simulink model "SEL_Model"  (R2022b)
settings: Solver=VariableStepAuto  StartTime=0.0  StopTime=10  RelTol=1e-3
model workspace (MAT data in the model file):
  QL = Simulink.Parameter
  QL.Value = 3000000
  QL.DataType = 'auto'
  QL.Complexity = 'real'
  QL.Dimensions = [1 1]
  RL = Simulink.Parameter
  RL.Value = 1560000000
  RL.DataType = 'auto'
  RL.Complexity = 'real'
  RL.Dimensions = [1 1]
  RQ = Simulink.Parameter
  RQ.Value = Simulink.data.Expression
  RQ.Value.ExpressionString = "RL/QL"
  RQ.DataType = 'auto'
  RQ.Complexity = 'real'
  RQ.Dimensions = -1
  Ts = Simulink.Parameter
  Ts.Value = 1e-07
  Ts.DataType = 'auto'
  Ts.Complexity = 'real'
  Ts.Dimensions = [1 1]
  a0 = Simulink.Parameter
  a0.Value = 1
  a0.DataType = 'auto'
  a0.Complexity = 'real'
  a0.Dimensions = [1 1]
  a1 = Simulink.Parameter
  a1.Value = -2
  a1.DataType = 'auto'
  a1.Complexity = 'real'
  a1.Dimensions = [1 1]
  a2 = Simulink.Parameter
  a2.Value = 1
  a2.DataType = 'auto'
  a2.Complexity = 'real'
  a2.Dimensions = [1 1]
  b0 = Simulink.Parameter
  b0.Value = -2.18e-09
  b0.DataType = 'auto'
  b0.Complexity = 'real'
  b0.Dimensions = [1 1]
  b1 = Simulink.Parameter
  b1.Value = -4.36e-09
  b1.DataType = 'auto'
  b1.Complexity = 'real'
  b1.Dimensions = [1 1]
  b2 = Simulink.Parameter
  b2.Value = -2.18e-09
  b2.DataType = 'auto'
  b2.Complexity = 'real'
  b2.Dimensions = [1 1]
  f0 = Simulink.Parameter
  f0.Value = 1300000000
  f0.DataType = 'auto'
  f0.Complexity = 'real'
  f0.Dimensions = [1 1]
  pi = Simulink.Parameter
  pi.Value = 3.1415926535
  pi.DataType = 'auto'
  pi.Complexity = 'real'
  pi.Dimensions = [1 1]
  w0 = Simulink.Parameter
  w0.Value = Simulink.data.Expression
  w0.Value.ExpressionString = "2*pi*390"
  w0.DataType = 'auto'
  w0.Complexity = 'real'
  w0.Dimensions = -1
  w_hbw = Simulink.Parameter
  w_hbw.Value = Simulink.data.Expression
  w_hbw.Value.ExpressionString = "2*pi*216"
  w_hbw.DataType = 'auto'
  w_hbw.Complexity = 'real'
  w_hbw.Dimensions = -1
settings Model: Creator=mliu  LastModifiedBy=mliu

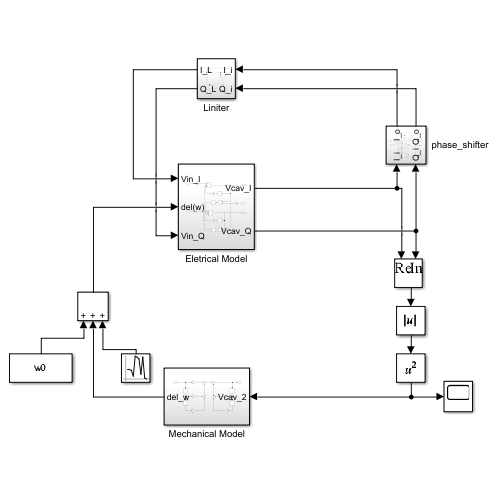
[thumbnail: Simulink's stored preview of the top-level diagram]
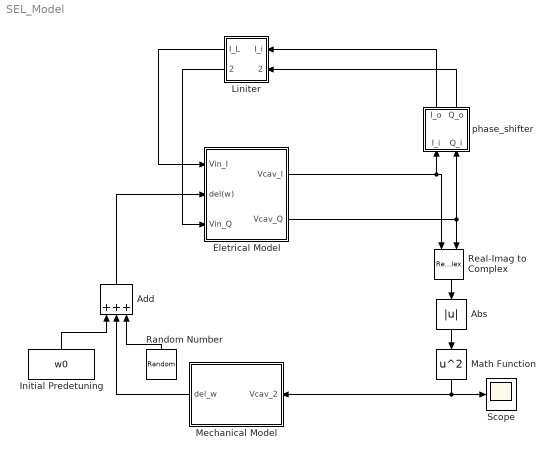
== system SEL_Model ==
  Abs : Abs  SaturateOnIntegerOverflow=off
  Add : Sum  Inputs=+++
  Eletrical Model : Subsystem
  Initial Predetuning : Constant  Value=w0
  Liniter : Subsystem
  Math Function : Math  Operator=square
  Mechanical Model : Subsystem
  Random Number : RandomNumber  SampleTime=0.1
  Real-Imag to Complex : RealImagToComplex
  Scope : Scope
  phase_shifter : Subsystem
  wires:
  Mechanical Model/1(del_w) -> Add/2
  Add/1 -> Eletrical Model/2(del(w))
  Initial Predetuning/1 -> Add/1
  Eletrical Model/1(Vcav_I) -> Real-Imag to Complex/1, phase_shifter/1(I_i)
  Eletrical Model/2(Vcav_Q) -> phase_shifter/2(Q_i), Real-Imag to Complex/2
  phase_shifter/1(I_o) -> Liniter/1(I_i)
  phase_shifter/2(Q_o) -> Liniter/2(Q_i)
  Liniter/2(Q_L) -> Eletrical Model/3(Vin_Q)
  Math Function/1 -> Scope/1, Mechanical Model/1(Vcav_2)
  Real-Imag to Complex/1 -> Abs/1
  Abs/1 -> Math Function/1
  Random Number/1 -> Add/3
  Liniter/1(I_L) -> Eletrical Model/1(Vin_I)

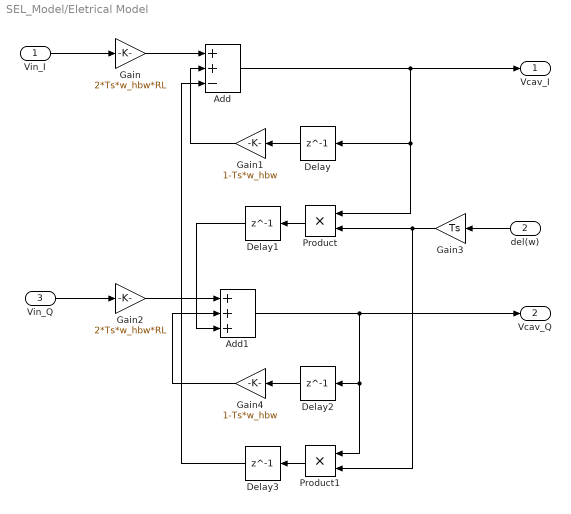
== system SEL_Model/Eletrical Model ==
  Vin_I : Inport
  del(w) : Inport  Port=2
  Vin_Q : Inport  Port=3
  Add : Sum  Inputs=++-
  Add1 : Sum  Inputs=+++
  Delay{,1..3} (4 alike) : Delay  DelayLength=1  InitialCondition=0
  Gain : Gain  Gain=2*Ts*w_hbw*RL
  Gain1 : Gain  Gain=1-Ts*w_hbw
  Gain2 : Gain  Gain=2*Ts*w_hbw*RL
  Gain3 : Gain  Gain=Ts
  Gain4 : Gain  Gain=1-Ts*w_hbw
  Product : Product
  Product1 : Product
  Vcav_I : Outport
  Vcav_Q : Outport  Port=2
  wires:
  Delay/1 -> Gain1/1
  Gain/1 -> Add/1
  Gain3/1 -> Product1/2, Product/2
  Add1/1 -> Vcav_Q/1, Product1/1, Delay2/1
  Add/1 -> Vcav_I/1, Product/1, Delay/1
  Delay1/1 -> Add1/3
  Product/1 -> Delay1/1
  Vin_Q/1 -> Gain2/1
  Vin_I/1 -> Gain/1
  Gain2/1 -> Add1/1
  Product1/1 -> Delay3/1
  Gain1/1 -> Add/2
  Delay2/1 -> Gain4/1
  Delay3/1 -> Add/3
  del(w)/1 -> Gain3/1
  Gain4/1 -> Add1/2

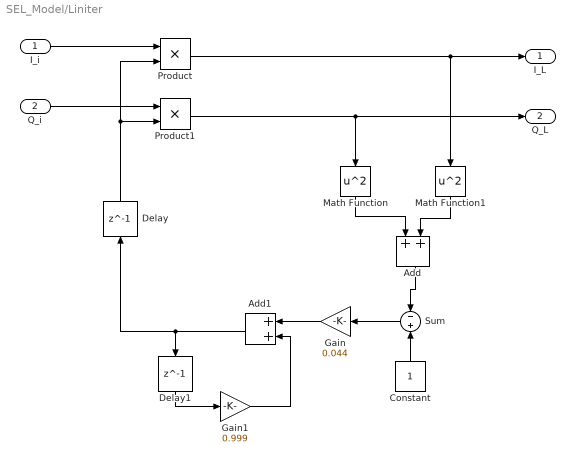
== system SEL_Model/Liniter ==
  I_i : Inport
  Q_i : Inport  Port=2
  Add : Sum
  Add1 : Sum
  Constant : Constant
  Delay : Delay  DelayLength=1  InitialCondition=0
  Delay1 : Delay  DelayLength=1  InitialCondition=0
  Gain : Gain  Gain=0.044
  Gain1 : Gain  Gain=0.999
  Math Function : Math  Operator=square
  Math Function1 : Math  Operator=square
  Product : Product
  Product1 : Product
  Sum : Sum  Inputs=-|+
  I_L : Outport
  Q_L : Outport  Port=2
  wires:
  Add/1 -> Sum/1
  Constant/1 -> Sum/2
  Sum/1 -> Gain/1
  Gain1/1 -> Add1/2
  Delay1/1 -> Gain1/1
  Add1/1 -> Delay1/1, Delay/1
  Product1/1 -> Q_L/1, Math Function/1
  Delay/1 -> Product1/2, Product/2
  Math Function/1 -> Add/1
  I_i/1 -> Product/1
  Gain/1 -> Add1/1
  Q_i/1 -> Product1/1
  Math Function1/1 -> Add/2
  Product/1 -> I_L/1, Math Function1/1

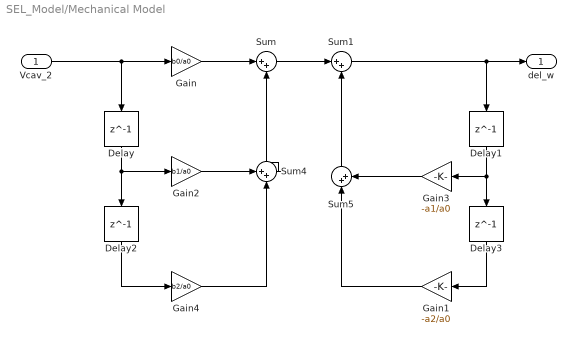
== system SEL_Model/Mechanical Model ==
  Vcav_2 : Inport
  Delay{,1..3} (4 alike) : Delay  DelayLength=1  InitialCondition=0
  Gain : Gain  Gain=b0/a0
  Gain1 : Gain  Gain=-a2/a0
  Gain2 : Gain  Gain=b1/a0
  Gain3 : Gain  Gain=-a1/a0
  Gain4 : Gain  Gain=b2/a0
  Sum{,1,4..5} (4 alike) : Sum  Inputs=|++
  del_w : Outport
  wires:
  Sum5/1 -> Sum1/2
  Gain3/1 -> Sum5/2
  Delay1/1 -> Gain3/1, Delay3/1
  Gain/1 -> Sum/1
  Gain2/1 -> Sum4/1
  Sum1/1 -> del_w/1, Delay1/1
  Sum4/1 -> Sum/2
  Sum/1 -> Sum1/1
  Vcav_2/1 -> Delay/1, Gain/1
  Gain1/1 -> Sum5/1
  Delay2/1 -> Gain4/1
  Gain4/1 -> Sum4/2
  Delay/1 -> Gain2/1, Delay2/1
  Delay3/1 -> Gain1/1

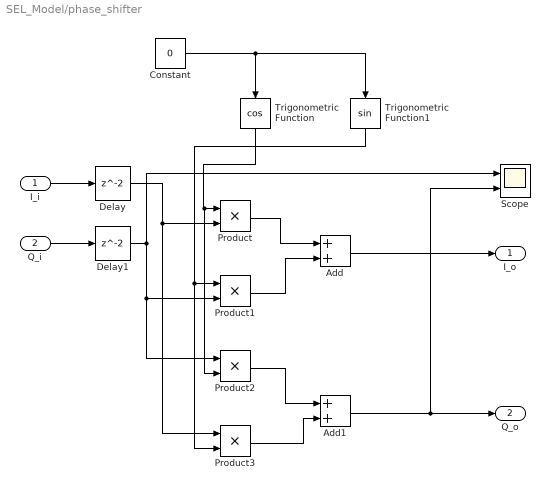
== system SEL_Model/phase_shifter ==
  I_i : Inport
  Q_i : Inport  Port=2
  Add : Sum
  Add1 : Sum
  Constant : Constant  Value=0
  Delay : Delay  InitialCondition=0
  Delay1 : Delay  InitialCondition=0
  Product{,1..3} (4 alike) : Product
  Scope : Scope  NumInputPorts=2
  Trigonometric Function : Trigonometry  Operator=cos
  Trigonometric Function1 : Trigonometry
  I_o : Outport
  Q_o : Outport  Port=2
  wires:
  Delay/1 -> Product3/1, Product/2
  Product1/1 -> Add/2
  Delay1/1 -> Scope/1, Product2/1, Product1/2
  Q_i/1 -> Delay1/1
  Add1/1 -> Q_o/1, Scope/2
  Product/1 -> Add/1
  Product3/1 -> Add1/2
  Product2/1 -> Add1/1
  Trigonometric Function/1 -> Product2/2, Product/1
  Constant/1 -> Trigonometric Function/1, Trigonometric Function1/1
  I_i/1 -> Delay/1
  Trigonometric Function1/1 -> Product3/2, Product1/1
  Add/1 -> I_o/1
